simulink library "ex"  (R2017b)
settings: Solver=VariableStepAuto  StartTime=0.0  StopTime=10.0  RelTol=1e-3
settings Model: Creator=MY  LastModifiedBy=MY

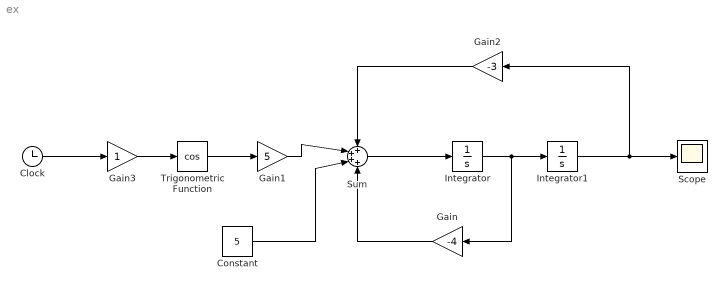
== system ex ==
  Clock : Clock
  Constant : Constant  Value=5
  Gain : Gain  Gain=-4
  Gain1 : Gain  Gain=5
  Gain2 : Gain  Gain=-3
  Gain3 : Gain
  Integrator : Integrator
  Integrator1 : Integrator
  Scope : Scope
  Sum : Sum  Inputs=++++
  Trigonometric Function : Trigonometry  Operator=cos
  wires:
  Integrator/1 -> Gain/1, Integrator1/1
  Sum/1 -> Integrator/1
  Constant/1 -> Sum/3
  Gain/1 -> Sum/4
  Trigonometric Function/1 -> Gain1/1
  Gain1/1 -> Sum/2
  Integrator1/1 -> Gain2/1, Scope/1
  Gain2/1 -> Sum/1
  Clock/1 -> Gain3/1
  Gain3/1 -> Trigonometric Function/1
